simulink model "formation_control_4N"  (R2021a)
settings: Solver=VariableStepAuto  StartTime=0.0  StopTime=T  RelTol=1e-3
undefined symbols (not defined in the file or in its folder): params
settings Model: Creator=gaeta  LastModifiedBy=giuse
settings SolverCC: AlgebraicLoopSolver=TrustRegion
settings DataIOCC: InitialState=initialCondition  LoadInitialState=on
settings DebuggingCC: SFMachineParentedDataDiag=warning

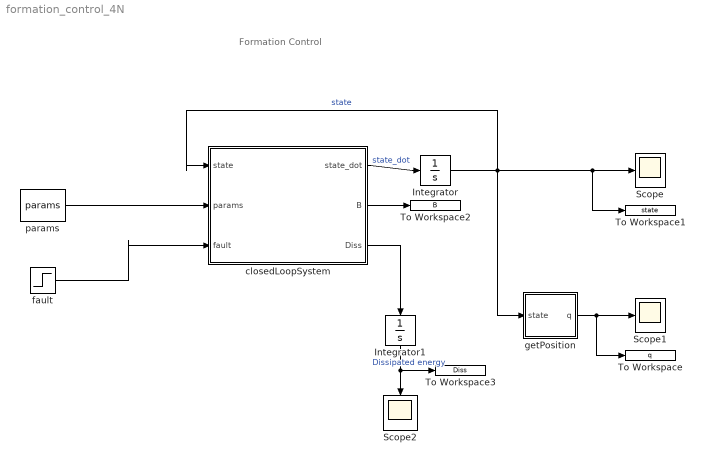
== system formation_control_4N ==
  note: Formation Control
  Integrator : Integrator
  Integrator1 : Integrator
  Scope : Scope
  Scope1 : Scope
  Scope2 : Scope
  To Workspace : ToWorkspace  VariableName=q  SaveFormat=Timeseries  SampleTime=-1
  To Workspace1 : ToWorkspace  VariableName=state  SaveFormat=Timeseries  SampleTime=-1
  To Workspace2 : ToWorkspace  VariableName=B  SaveFormat=Timeseries  SampleTime=-1
  To Workspace3 : ToWorkspace  VariableName=Diss  SaveFormat=Timeseries  SampleTime=-1
  closedLoopSystem : MATLAB Function  TreatAsAtomicUnit=on
  fault : Step  Time=15  After=4  SampleTime=0
  getPosition : Subsystem
  params : Constant  Value=params  OutDataTypeStr=Bus: params_bus
  wires:
  params/1 -> closedLoopSystem/2(params)
  Integrator/1 -> closedLoopSystem/1(state), Scope/1, To Workspace1/1, getPosition/1(state)  "state"
  closedLoopSystem/1(state_dot) -> Integrator/1  "state_dot"
  getPosition/1(q) -> Scope1/1, To Workspace/1
  fault/1 -> closedLoopSystem/3(fault)
  closedLoopSystem/2(B) -> To Workspace2/1
  closedLoopSystem/3(Diss) -> Integrator1/1
  Integrator1/1 -> Scope2/1, To Workspace3/1  "Dissipated energy"

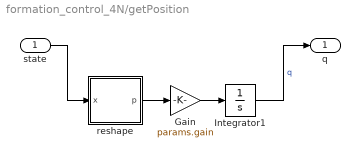
== system formation_control_4N/getPosition ==
  state : Inport
  Gain : Gain  Gain=params.gain
  Integrator1 : Integrator
  reshape : MATLAB Function  TreatAsAtomicUnit=on
  q : Outport
  wires:
  state/1 -> reshape/1(x)
  reshape/1(p) -> Gain/1
  Gain/1 -> Integrator1/1
  Integrator1/1 -> q/1  "q"

== matlab function formation_control_4N/closedLoopSystem ==
  data: state input size=3*(params.N+params.E); state_dot output size=3*(params.N+params.E); params input; B output; fault input; Diss output
function [state_dot,B,Diss] = closedLoopSystem(state, params, fault)
    n = 3;                      % task space
    N = params.N;               % number of robots
    
    p = state(1:n*N);           % robots momenta
    m = params.m;               % robots masses
    M = zeros(n*N, n*N);      	% inertia matrix
    d = params.d;               % frict. coeff
    D = zeros(n*N, n*N);        % system dissipation matrix
    for i = 1:N
        M(n*i-n+1:n*i, n*i-n+1:n*i) = eye(n).*m(i);
        D(n*i-n+1:n*i, n*i-n+1:n*i) = eye(n).*d(i);
    end
    
    E = params.E;               % number of edges
    if(fault && ~params.fault_occurred)
        params.fault_occurred = 1;  % flag on
        %faulted_robot = int8(round(fault));    % does not work (why?)
        faulted_robot = 4;
        params.B = faultHandler(params.B, params.Bfull, faulted_robot);
    end
    B = params.B;
    Bcl = kron(params.B,eye(n));	% closed-loop incidence matrix    

    z = state(n*N+1:n*(N+E));	% edges lengths
    z_des = params.z_des;       % desired edges lengths
    dc = params.dc;             % robots dissipations
    Dc = zeros(n*E, n*E);       % controller dissipation matrix
    kc = params.kc;             % constant springs
    Kc = zeros(n*E, n*E);       % constant spring matrix
    for j = 1:E
        Dc(n*j-n+1:n*j, n*j-n+1:n*j) = eye(n).*dc(j);
        Kc(n*j-n+1:n*j, n*j-n+1:n*j) = eye(n).*kc(j);
    end
    
    gamma = params.gamma;
    
    Diss = p.'*(inv(M.')*D*inv(M))*p;   % energy dissipation
    Fe = -Bcl * Kc*(z-z_des);           % external forces (control action)
    Fa = -(Bcl*Dc*Bcl.')*(M^(-1)*p);    % interaction (coupling) forces
    
    %{
    Fa_ij = ??;
    wz_ij = -gamma*Fa_ij*t_i^2 - gamma*Fa_ij*t_j^2;
    wt_ij = -gamma*(Fa_ij.'*Fa_ij)*t_i;
    wt_ij = -gamma*(Fa_ij.'*Fa_ij)*t_j;
    dt_i = (1/t_i)*Diss + wt_ij;
    %}
    
    p_dot = Fa + Fe - D*(M^(-1)*p);
    z_dot = Bcl.'*(M^(-1)*p);
    state_dot = [p_dot; z_dot];
   
end


function B = faultHandler(B, Bfull, fault)

    % split 
    if(fault==1)
        disp("leader cannot be faulted by hypothesis");
    else
        z = zeros(size(B,1),2);
        B = [B(:, 1:fault-2), z, B(:, fault+1:size(B,2))];
        B(fault,:) = zeros(1, size(B,2));
    end
    
    % join
    N = size(B,1);
    if(fault==N)
        r1 = fault-1;
        r2 = 1;
    else
        r1 = fault-1;
        r2 = fault+1;
    end
	for e = 1:size(Bfull,2)
        if( (Bfull(r1,e)==1 && Bfull(r2,e)==-1) || (Bfull(r1,e)==-1 && Bfull(r2,e)==1) )
            B(:,e) = Bfull(:,e);
        end
	end
end



%

== matlab function formation_control_4N/getPosition/reshape ==
  data: p output size=params.N*3; x input
function p = reshape(x)
    N = 4; % number of robots
    p = x(1:3*N);
end




%
